simulink model "CaracterizacionMotores"  (R2022b)
settings: Solver=FixedStepDiscrete  StartTime=0.0  StopTime=10  FixedStep=0.01  RelTol=1e-3  EnableMultiTasking=on
libraries: SignalEditorBlockLib x1
settings Model: ExtModeTrigDuration=2  Creator=Usuario  LastModifiedBy=Usuario
settings SolverCC: AutoInsertRateTranBlk=on
settings OptimizationCC: ReuseModelBlockBuffer=on  EnhancedBackFolding=on  PassReuseOutputArgsAs=Individual arguments  ZeroExternalMemoryAtStartup=off  ZeroInternalMemoryAtStartup=off  MaxStackSize=64  OptimizeBlockOrder=speed  DifferentSizesBufferReuse=on  OptimizationCustomize=off  EfficientTunableParamExpr=on
settings DebuggingCC: ParameterTunabilityLossMsg=error
settings HardwareCC: ProdBitPerInt=16  ProdBitPerPointer=16  ProdBitPerSizeT=16  ProdBitPerPtrDiffT=16  ProdLargestAtomicFloat=None  ProdWordSize=8  ProdHWDeviceType=Atmel->AVR  UseEmbeddedCoderFeatures=off  UseSimulinkCoderFeatures=off
settings SFSimCC: MATLABDynamicMemAlloc=off
settings RTWCC: Description=Embedded Coder  SystemTargetFile=ert.tlc  HardwareBoard=Arduino Mega 2560  TLCOptions=-aInlineSetEventsForThisBaseRateFcn=TLC_FALSE -aSuppressMultiTaskScheduler=TLC_FALSE -aRateBasedStepFcn=1  TemplateMakefile=ert_default_tmf  Toolchain=Arduino AVR  BuildConfiguration=Faster Runs  GPUComputeCapability=5.0
settings CodeAppCC: ForceParamTrailComments=on  IgnoreCustomStorageClasses=off  OperatorAnnotations=on  SimulinkDataObjDesc=on  SFDataObjDesc=on  InsertBlockDesc=on
settings ERTTargetCC: SupportContinuousTime=on  SupportNonInlinedSFcns=on  SupportVariableSizeSignals=on  ExtModeTransport=3  ExtModeStaticAlloc=on  ExtModeAutomaticAllocSize=off  ExtModeStaticAllocSize=2048  ExtModeMexFile=ext_xcp  ExtModeIntrfLevel=Level2 - Open
settings SettingsController: UseSoCProfilerForTargets=0

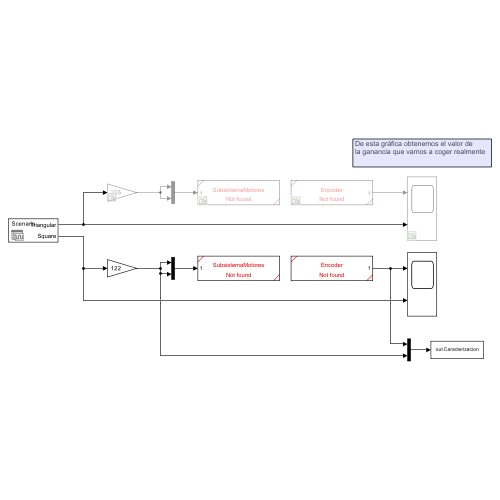
[thumbnail: Simulink's stored preview of the top-level diagram]
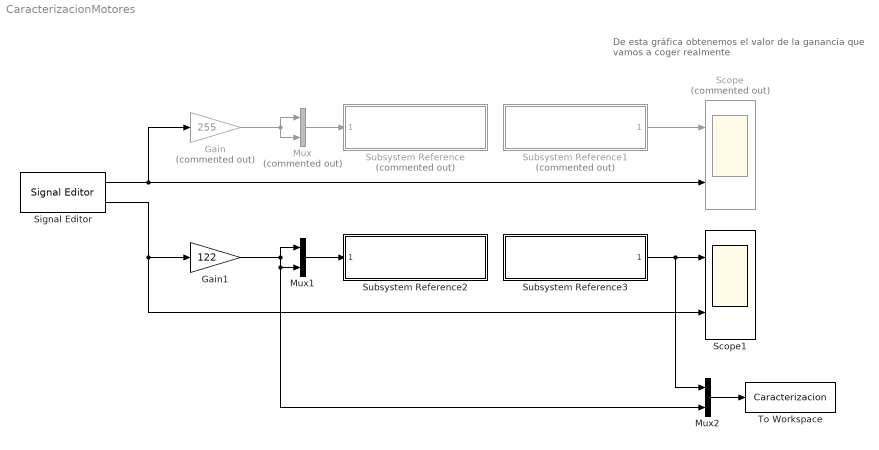
== system CaracterizacionMotores ==
  note: De esta gráfica obtenemos el valor de
      | la ganancia que vamos a coger realmente
  Gain : Gain  Commented=on  Gain=255
  Gain1 : Gain  Gain=122
  Mux : Mux  Commented=on  Inputs=2
  Mux1 : Mux  Inputs=2
  Mux2 : Mux  Inputs=2
  Scope : Scope  Commented=on  NumInputPorts=2
  Scope1 : Scope  NumInputPorts=2
  Signal Editor : SignalEditorBlockLib/Signal Editor  FileName=C:\Users\Usuario\Desktop\prueba2\lib\Ssignal.mat  ActiveScenario=Scenario  ActiveSignal=Triangular  IsBus=off  OutputBusObjectStr=Bus: BusObject  SampleTime=0  ZeroCross=off  OutputAfterFinalValue=Setting to zero  Unit=inherit  PreserveSignalName=on
  Subsystem Reference : Subsystem  Commented=on  ReferencedSubsystem=SubsistemaMotores
  Subsystem Reference1 : Subsystem  Commented=on  ReferencedSubsystem=Encoder
  Subsystem Reference2 : Subsystem  ReferencedSubsystem=SubsistemaMotores
  Subsystem Reference3 : Subsystem  ReferencedSubsystem=Encoder
  To Workspace : ToWorkspace  VariableName=Caracterizacion  SampleTime=0.01
      settings: Save2DSignal=2-D array (concatenate along first dimension)
  wires:
  Signal Editor/1 -> Gain/1, Scope/2
  Mux/1 -> Subsystem Reference/1
  Gain/1 -> Mux/1, Mux/2
  Subsystem Reference1/1 -> Scope/1
  Mux1/1 -> Subsystem Reference2/1
  Signal Editor/2 -> Scope1/2, Gain1/1
  Gain1/1 -> Mux1/1, Mux1/2, Mux2/2
  Subsystem Reference3/1 -> Mux2/1, Scope1/1
  Mux2/1 -> To Workspace/1
